simulink model "Switchexp2"  (R2015b)
settings: Solver=VariableStepAuto  StartTime=0.0  StopTime=10.0  RelTol=1e-3
libraries: dspsrcs4 x1
settings Model: Creator=LUBO  LastModifiedBy=LUBO

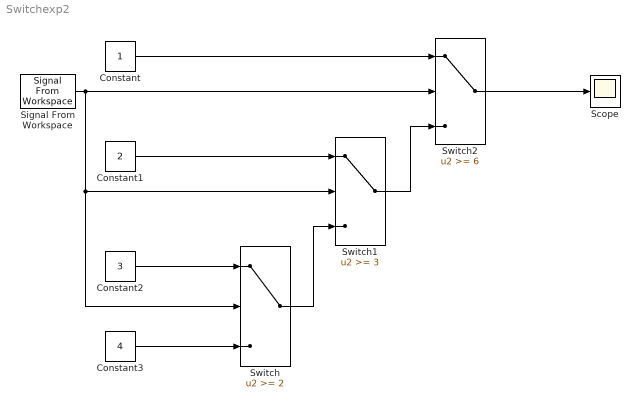
== system Switchexp2 ==
  Constant : Constant
  Constant1 : Constant  Value=2
  Constant2 : Constant  Value=3
  Constant3 : Constant  Value=4
  Scope : Scope
  Signal From Workspace : dspsrcs4/Signal From Workspace  X=1:10  Ts=1  nsamps=1  OutputAfterFinalValue=Setting to zero  ignoreOrWarnInputAndFrameLengths=off  OutputFrames=off
  Switch : Switch  Threshold=2  ZeroCross=off
  Switch1 : Switch  Threshold=3
  Switch2 : Switch  Threshold=6
  wires:
  Constant/1 -> Switch2/1
  Constant1/1 -> Switch1/1
  Switch1/1 -> Switch2/3
  Switch/1 -> Switch1/3
  Constant3/1 -> Switch/3
  Constant2/1 -> Switch/1
  Switch2/1 -> Scope/1
  Signal From Workspace/1 -> Switch/2, Switch1/2, Switch2/2
